simulink model "DepartPiste2"  (R2021a)
settings: Solver=FixedStepDiscrete  StartTime=0.0  StopTime=8.75  RelTol=1e-3  EnableMultiTasking=on
libraries: dsparch4 x5, dspsrcs4 x2, dspsigops x1, commanapbnd3 x1
settings Model: Creator=sebastienroy  LastModifiedBy=roys2121
settings SolverCC: AlgebraicLoopSolver=TrustRegion
settings DataIOCC: LimitDataPoints=on  SaveFormat=Array  ReturnWorkspaceOutputs=off
settings OptimizationCC: LifeSpan=inf
settings DebuggingCC: UnderspecifiedInitializationDetection=Classic  MergeDetectMultiDrivingBlocksExec=none  SolverPrmCheckMsg=warning  StateNameClashWarn=warning  SFUnexpectedBacktrackingDiag=warning  SFNoUnconditionalDefaultTransitionDiag=warning  SFExecutionAtInitializationDiag=none  SFMachineParentedDataDiag=warning  ArithmeticOperatorsInVariantConditions=warning
settings HardwareCC: ProdBitPerPointer=32  ProdBitPerSizeT=32  ProdBitPerPtrDiffT=32  ProdLargestAtomicFloat=None  ProdIntDivRoundTo=Undefined  ProdEndianess=Unspecified  ProdWordSize=32  ProdHWDeviceType=32-bit Generic
settings ModelReferenceCC: PropagateSignalLabelsOutOfModel=off
settings SFSimCC: SimUseLocalCustomCode=off  CustomCodeUndefinedFunction=UseInterfaceOnly
settings RTWCC: RTWUseLocalCustomCode=off
settings CodeAppCC: StateflowObjectComments=on
settings GRTTargetCC: TargetLangStandard=C89/C90 (ANSI)
settings ConfigComp: CovMetricSettings=dw  CovSaveCumulativeToWorkspaceVar=on  CovSaveSingleToWorkspaceVar=on  CovExternalEMLEnable=off

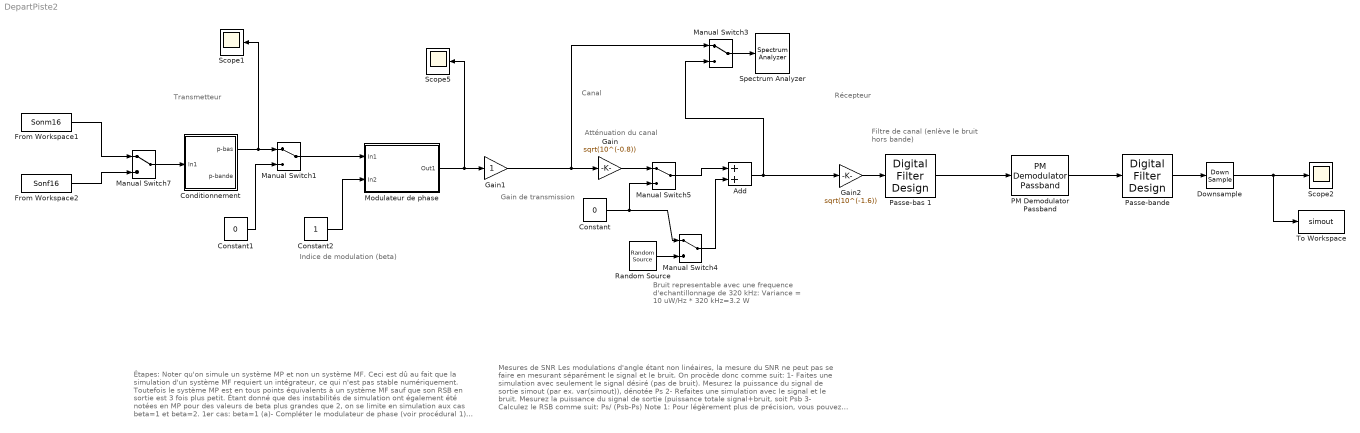
== system DepartPiste2 ==
  note: Indice de modulation (beta)
  note: Filtre de canal
      | (enlève le bruit hors bande)
  note: Récepteur
  note: Canal
  note: Transmetteur
  note: Atténuation du canal
  note: Gain de transmission
  note: Bruit representable avec une frequence
      | d'echantillonnage de 320 kHz:
      | Variance = 10 uW/Hz * 320 kHz=3.2 W
  note: Étapes:
      |
      | Noter qu'on simule un système MP et non un système MF. Ceci est dû au fait que la simulation d'un système MF requiert un intégrateur, ce qui n'est pas stable numériquement. Toutefois le système MP est en tous points équivalents à un système MF sauf que son RSB en sortie est 3 fois plus petit. Étant donné que des instabilités de simulation ont également été notées en MP pour des valeurs de beta plus grandes que 2, on se limite en simulation aux cas beta=1 et beta=2.
      |
      | 1er cas: beta=1
      | (a)- Compléter le modulateur de phase (voir procédural 1)
      | (b)- Trouver le bon gain de transmission et insérer-le dans le bloc correspondant
      | (c)- Vérifier que le système fonctionne
      | (d)- Mesurer le RSB (selon la procédure à droite) et comparer avec la théorie pour beta=1 (voir note 2 à droite).
      |
      | 2e cas: beta=2
      | (a)- Déterminer la largeur de bande B_T du signal modulé avec beta=2
      | (b)- Choisir une fréquence de porteuse pour que le signal modulé occupe la bande entre 0 et B_T
      | (c)- Modifier le modulateur de phase avec le nouveau beta et la nouvelle fréquence porteuse (dans les oscillateurs)
      | (c)- Modifier le démodulateur de phase avec le nouveau beta et la nouvelle fréquence porteuse (ouvrir le bloc)
      | (d)- Modifier le filtre canal au récepteur pour que sa fréquence de coupure soit égale à B_T
      | (e)- Tester le système et mesurer le RSB (selon la procédure à droite); comparer avec la théorie pour beta=2.
  note: Mesures de SNR
      |
      | Les modulations d'angle étant non linéaires, la mesure du SNR ne peut pas se faire
      | en mesurant séparément le signal et le bruit. On procède donc comme suit:
      | 1- Faites une simulation avec seulement le signal désiré (pas de bruit). Mesurez la puissance du signal de sortie simout (par ex. var(simout)), dénotée Ps
      | 2- Refaites une simulation avec le signal et le bruit. Mesurez la puissance du signal de sortie (puissance totale signal+bruit, soit Psb
      | 3- Calculez le RSB comme suit: Ps/ (Psb-Ps)
      |
      | Note 1: Pour légèrement plus de précision, vous pouvez éliminer le transitoire au début du signal de sortie en prenant var(simout(400:140001)).
      |
      | Note 2: Il est normal de trouver un RSB_o plus bas (jusqu'à 50%) en simulation à cause des imperfections de la simulation numérique. Par ailleurs, l'écart entre le RSB théorique et le RSB mesuré en simulation augmente lorsque le RSB est faible. Ceci est normal, car les effets non-linéaires augmentent et la formule théorique n'en tient pas compte. En effet, c'est une formule basée sur un modèle linéaire, donc pas entièrement exacte.
  Add : Sum
  Conditionnement : Subsystem
  Constant : Constant  Value=0
  Constant1 : Constant  Value=0
  Constant2 : Constant
  Downsample : DownSample  N=20  RateOptions=Allow multirate processing
  From Workspace1 : FromWorkspace  VariableName=Sonm16  SampleTime=1/16000  Interpolate=off  OutputAfterFinalValue=Setting to zero
  From Workspace2 : FromWorkspace  VariableName=Sonf16  SampleTime=1/16000  Interpolate=off  OutputAfterFinalValue=Setting to zero
  Gain : Gain  Gain=sqrt(10^(-0.8))
  Gain1 : Gain
  Gain2 : Gain  Gain=sqrt(10^(-1.6))
  Manual Switch{1,3..5,7} (5 alike) : ManualSwitch
  Modulateur de phase : Subsystem
  PM Demodulator Passband : commanapbnd3/PM Demodulator Passband  Fc=6800  Ph=0  Kc=1  Ho=100
      settings: SourceProductBaseCode=CM
  Passe-bande : dsparch4/Digital Filter Design  mwdsp_browser_bugfix_var=off
  Passe-bas 1 : dsparch4/Digital Filter Design  mwdsp_browser_bugfix_var=off
  Random Source : dspsrcs4/Random Source  SrcType=Gaussian  NormMethod=Ziggurat  CltLength=12  MinVal=0  MaxVal=1  MeanVal=0  VarVal=3.2  RepMode=Specify seed  rawSeed=2  IsInherit=on  SampMode=Discrete  SampTime=1  SampFrame=1  DataType=Double  OutComplex=Real  OutputFrames=on
  Scope1 : Scope
  Scope2 : Scope
  Scope5 : Scope
  Spectrum Analyzer : SpectrumAnalyzer
  To Workspace : ToWorkspace  VariableName=simout  SampleTime=-1
      settings: Save2DSignal=2-D array (concatenate along first dimension)
  wires:
  Manual Switch3/1 -> Spectrum Analyzer/1
  Gain1/1 -> Gain/1, Manual Switch3/1
  Random Source/1 -> Manual Switch4/2
  Manual Switch4/1 -> Add/2
  Gain/1 -> Manual Switch5/1
  Manual Switch5/1 -> Add/1
  Constant/1 -> Manual Switch4/1, Manual Switch5/2
  Conditionnement/1(p-bas) -> Scope1/1, Manual Switch1/1
  Modulateur de phase/1(Out1) -> Scope5/1, Gain1/1
  Add/1 -> Gain2/1, Manual Switch3/2
  Constant1/1 -> Manual Switch1/2
  Downsample/1 -> To Workspace/1, Scope2/1
  Gain2/1 -> Passe-bas 1/1
  Manual Switch1/1 -> Modulateur de phase/1(In1)
  Passe-bas 1/1 -> PM Demodulator Passband/1
  Manual Switch7/1 -> Conditionnement/1(In1)
  From Workspace2/1 -> Manual Switch7/2
  From Workspace1/1 -> Manual Switch7/1
  Constant2/1 -> Modulateur de phase/2(In2)
  Passe-bande/1 -> Downsample/1
  PM Demodulator Passband/1 -> Passe-bande/1

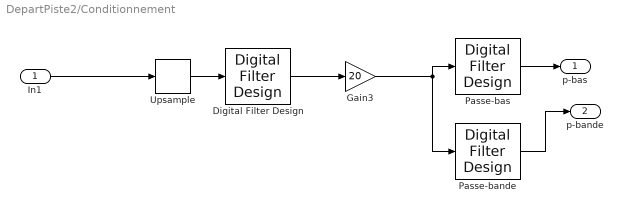
== system DepartPiste2/Conditionnement ==
  In1 : Inport
  Digital Filter Design : dsparch4/Digital Filter Design  mwdsp_browser_bugfix_var=off
  Gain3 : Gain  Gain=20
  Passe-bande : dsparch4/Digital Filter Design  mwdsp_browser_bugfix_var=off
  "Passe-bas " : dsparch4/Digital Filter Design  mwdsp_browser_bugfix_var=off
  Upsample : dspsigops/Upsample  N=20  phase=0  RateOptions=Allow multirate processing  ic=0  mode=Unused parameter value
  p-bas : Outport
  p-bande : Outport  Port=2
  wires:
  Upsample/1 -> Digital Filter Design/1
  "Passe-bas "/1 -> p-bas/1
  Digital Filter Design/1 -> Gain3/1
  Passe-bande/1 -> p-bande/1
  Gain3/1 -> "Passe-bas "/1, Passe-bande/1
  In1/1 -> Upsample/1

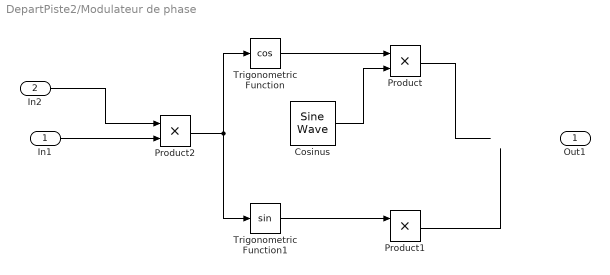
== system DepartPiste2/Modulateur de phase ==
  In1 : Inport
  In2 : Inport  Port=2
  Cosinus : dspsrcs4/Sine Wave  Amplitude=1  Frequency=6800  Phase=0  SampleMode=Discrete  OutComplex=Real  CompMethod=Trigonometric fcn  TableSize=Speed  SampleTime=1/320000  SamplesPerFrame=1  ResetState=Restart at time zero  OutputFrames=off  dataType=double  wordLen=16  udDataType=sfix(16)  fracBitsMode=Best precision  numFracBits=15  OutDataTypeStr=double  LastOutDataTypeStr=double
  Product : Product
  Product1 : Product
  Product2 : Product
  Trigonometric Function : Trigonometry  Operator=cos
  Trigonometric Function1 : Trigonometry
  Out1 : Outport
  wires:
  In1/1 -> Product2/2
  Cosinus/1 -> Product/2
  ? -> Out1/1
  Product/1 -> ?
  Product2/1 -> Trigonometric Function1/1, Trigonometric Function/1
  Trigonometric Function/1 -> Product/1
  Product1/1 -> ?
  In2/1 -> Product2/1
  Trigonometric Function1/1 -> Product1/1
  ? -> Product1/2
